simulink model "Voltage_Vector_with_script_fianl"  (R2024b)
settings: Solver=FixedStepAuto  StartTime=0.0  StopTime=0.5  FixedStep=1e-5  RelTol=1e-3
model workspace (MAT data in the model file):
  Cap = 0.004
  FL = 0.025
  Indcut = 0.005
  Initial_Voltage = 125
  R_Load = 1000
  V_dc = 300
  Vd = 125
  Vl = 400
  c = 125
  cap = 7.07e-05
  f_o = 50
  f_s = 5000
libraries: spsIGBTDiodeLib x72, spsSeriesRLCBranchLib x48, spsMultimeterLib x9, spsRMSLib x7, spsThreePhaseBreakerLib x6, spsTHDLib x6, spsThreePhaseSeriesRLCLoadLib x4, spsGroundLib x3, spsCurrentMeasurementLib x2, spsDCVoltageSourceLib x2, spsThreePhaseVIMeasurementLib x2, slpidlib x1
(part 2 of 3)

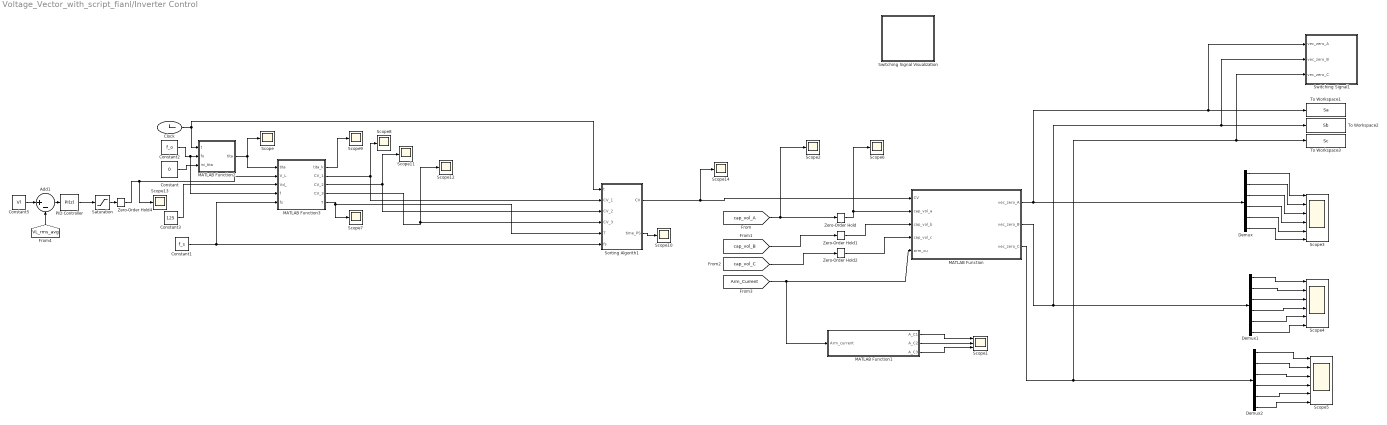
== system Voltage_Vector_with_script_fianl/Inverter Control ==
  Add1 : Sum  Inputs=|+-
  Clock : Clock
  Constant : Constant  Value=0
  Constant1 : Constant  Value=f_s
  Constant2 : Constant  Value=f_o
  Constant3 : Constant  Value=125
  Constant5 : Constant  Value=Vl
  Demux : Demux  Outputs=6
  Demux1 : Demux  Outputs=6
  Demux2 : Demux  Outputs=6
  MATLAB Function : MATLAB Function  TreatAsAtomicUnit=on
  MATLAB Function1 : MATLAB Function  TreatAsAtomicUnit=on
  MATLAB Function2 : MATLAB Function  TreatAsAtomicUnit=on
  MATLAB Function3 : MATLAB Function  TreatAsAtomicUnit=on
  PID Controller : slpidlib/PID Controller  Controller=PI  Form=Parallel  TimeDomain=Discrete-time  UseExternalTs=off  SampleTime=-1  IntegratorMethod=Forward Euler  FilterMethod=Forward Euler  ControllerParametersSource=internal  P=9  I=80  UseKiTs=off  D=0  UseExternalDerivativeSource=off  N=100  UseFilter=on  TunerSelectOption=Transfer Function Based (PID Tuner App)  InitialConditionSource=internal  InitialConditionForIntegrator=0  InitialConditionForFilter=0  DifferentiatorICPrevScaledInput=0  ExternalReset=none  TrackingMode=off  Kt=1  LimitOutput=off  SatLimitsSource=internal  UpperSaturationLimit=inf  LowerSaturationLimit=-inf  LinearizeAsGain=on  AntiWindupMode=none  Kb=1  LimitIntegrator=off  UpperIntegratorSaturationLimit=inf  LowerIntegratorSaturationLimit=-inf  POutMin=[]  POutMax=[]  IOutMin=[]  IOutMax=[]  DOutMin=[]  DOutMax=[]  NOutMin=[]  NOutMax=[]  SumOutMin=[]  SumOutMax=[]  SaturationOutMin=[]  SaturationOutMax=[]  PParamMin=[]  PParamMax=[]  IParamMin=[]  IParamMax=[]  DParamMin=[]  DParamMax=[]  NParamMin=[]  NParamMax=[]  KbParamMin=[]  KbParamMax=[]  KtParamMin=[]  KtParamMax=[]  KbOutMin=[]  KbOutMax=[]  KtOutMin=[]  KtOutMax=[]  IntegratorOutMin=[]  IntegratorOutMax=[]  FilterOutMin=[]  FilterOutMax=[]  SumI1OutMin=[]  SumI1OutMax=[]  SumI2OutMin=[]  SumI2OutMax=[]  SumI3OutMin=[]  SumI3OutMax=[]  SumI4OutMin=[]  SumI4OutMax=[]  SumDOutMin=[]  SumDOutMax=[]  DifferentiatorOutMin=[]  DifferentiatorOutMax=[]  FilterDiffOutCoefMin=[]  FilterDiffOutCoefMax=[]  ReciprocalOutMin=[]  ReciprocalOutMax=[]  SumDenOutMin=[]  SumDenOutMax=[]  SumNumOutMin=[]  SumNumOutMax=[]  DivideOutMin=[]  DivideOutMax=[]  UdiffTsProdOutMin=[]  UdiffTsProdOutMax=[]  NTsProdOutMin=[]  NTsProdOutMax=[]  UintegralTsProdOutMin=[]  UintegralTsProdOutMax=[]  UngainTsProdOutMin=[]  UngainTsProdOutMax=[]  ClampingZeroOutDataTypeStr=Inherit: Inherit via back propagation  ClampingZeroOutMin=[]  ClampingZeroOutMax=[]  FilterDenConstantOutDataTypeStr=Inherit: Inherit via back propagation  FilterDenConstantOutMin=[]  FilterDenConstantOutMax=[]  PCopyOutDataTypeStr=Inherit: Inherit via back propagation  PCopyOutMin=[]  PCopyOutMax=[]  NCopyOutDataTypeStr=Inherit: Inherit via back propagation  NCopyOutMin=[]  NCopyOutMax=[]  IntegratorContinuousStateAttributes=''  IntegratorStateMustResolveToSignalObject=off  IntegratorRTWStateStorageClass=Auto  FilterContinuousStateAttributes=''  FilterStateMustResolveToSignalObject=off  FilterRTWStateStorageClass=Auto  ParallelPVariant=InternalParameters  IdealPVariant=Disabled  IVariant=InternalParameters  DVariant=Disabled  IntegratorVariant=Discrete  SatVariant=Disabled  AWVariant=Passthrough  PCopyVariant=Disabled  TRVariant=Disabled  FdbkBlocksVariant=Forward  IdealPFdbkVariant=Disabled  SatFdbkVariant=Disabled  DerivativeFilterVariant=Disabled  NVariant=Disabled  NCopyVariant=Disabled_SignalSpec  FilterICVariant=Disabled  IntegratorICVariant=InternalICs  ExternalResetVariant=Disabled  TRSumVariant=Passthrough  SumFdbkVariant=Disabled  SumVariant=Sum_PI  TsampFilterVariant=InternalTs  TsampNgainVariant=Passthrough  TsampIntegralVariant=Disabled_SignalSpec  ExternalSaturationOutDataTypeStr=Inherit: Same as second input  DerivativeSourceVariant=Disabled  PreIntVariant=InternalPreInt
  Saturation : Saturate  UpperLimit=450  LowerLimit=350
  Scope{,2,6..14} (11 alike) : Scope
  Scope1 : Scope  NumInputPorts=3
  Scope3 : Scope  NumInputPorts=6
  Scope4 : Scope  NumInputPorts=6
  Scope5 : Scope  NumInputPorts=6
  Sorting Algorith1 : MATLAB Function  TreatAsAtomicUnit=on
  Switching Signal Visualization : Subsystem
  Switching Signal1 : Subsystem
  To Workspace1 : ToWorkspace  VariableName=Sa  SaveFormat=Timeseries  SampleTime=-1
      settings: Decimation=10
  To Workspace2 : ToWorkspace  VariableName=Sb  SaveFormat=Timeseries  SampleTime=-1
  To Workspace3 : ToWorkspace  VariableName=Sc  SaveFormat=Timeseries  SampleTime=-1
  Zero-Order Hold{,1..2,4} (4 alike) : ZeroOrderHold  SampleTime=1/5000
  wires:
  [cap_vol_A] -> Zero-Order Hold/1, Scope2/1
  [Arm_Current] -> MATLAB Function/5(arm_cu), MATLAB Function1/1(Arm_current)
  MATLAB Function1/1(A_C1) -> Scope1/1
  MATLAB Function1/2(A_C2) -> Scope1/2
  MATLAB Function1/3(A_C3) -> Scope1/3
  Demux2/1 -> Scope5/1
  Demux2/6 -> Scope5/6
  Demux2/2 -> Scope5/2
  Demux2/3 -> Scope5/3
  Demux2/4 -> Scope5/4
  Demux2/5 -> Scope5/5
  Demux1/1 -> Scope4/1
  Demux1/6 -> Scope4/6
  Demux1/2 -> Scope4/2
  Demux1/3 -> Scope4/3
  Demux1/4 -> Scope4/4
  Demux1/5 -> Scope4/5
  MATLAB Function/2(vec_zero_B) -> Switching Signal1/2(vec_zero_B), To Workspace2/1, Demux1/1
  Demux/6 -> Scope3/6
  Demux/5 -> Scope3/5
  Demux/4 -> Scope3/4
  Demux/3 -> Scope3/3
  Demux/2 -> Scope3/2
  Demux/1 -> Scope3/1
  MATLAB Function/1(vec_zero_A) -> Switching Signal1/1(vec_zero_A), To Workspace1/1, Demux/1
  MATLAB Function/3(vec_zero_C) -> Switching Signal1/3(vec_zero_C), To Workspace3/1, Demux2/1
  Zero-Order Hold/1 -> Scope6/1, MATLAB Function/2(cap_vol_a)
  [cap_vol_B] -> Zero-Order Hold1/1
  Zero-Order Hold1/1 -> MATLAB Function/3(cap_vol_b)
  [cap_vol_C] -> Zero-Order Hold2/1
  Zero-Order Hold2/1 -> MATLAB Function/4(cap_vol_c)
  MATLAB Function3/4(CV_3) -> Scope12/1, Sorting Algorith1/4(CV_3)
  MATLAB Function3/3(CV_2) -> Scope11/1, Sorting Algorith1/3(CV_2)
  MATLAB Function3/5(T) -> Scope7/1, Sorting Algorith1/5(T)
  MATLAB Function3/1(tita_k) -> Scope9/1
  Constant2/1 -> MATLAB Function3/4(f), MATLAB Function2/2(fo)
  MATLAB Function2/1(tita) -> MATLAB Function3/1(tita), Scope/1
  Constant/1 -> MATLAB Function2/3(ini_tita)
  MATLAB Function3/2(CV_1) -> Scope8/1, Sorting Algorith1/2(CV_1)
  Clock/1 -> MATLAB Function2/1(t), Sorting Algorith1/1(t)
  Sorting Algorith1/1(CV) -> Scope14/1, MATLAB Function/1(CV)
  Sorting Algorith1/2(time_PS) -> Scope10/1
  Constant1/1 -> MATLAB Function3/5(fs), Sorting Algorith1/6(fs)
  Constant3/1 -> MATLAB Function3/3(Vd_)
  Constant5/1 -> Add1/1
  [VL_rms_avg] -> Add1/2
  Add1/1 -> PID Controller/1
  PID Controller/1 -> Saturation/1
  Saturation/1 -> Zero-Order Hold4/1
  Zero-Order Hold4/1 -> Scope13/1, MATLAB Function3/2(V_L)

== system Voltage_Vector_with_script_fianl/LC Filter ==
  Ground : spsGroundLib/Ground  LConnTagsString=a
  Series RLC Branch : spsSeriesRLCBranchLib/Series RLC Branch  LConnTagsString=__new0  RConnTagsString=__new0  BranchType=L  Resistance=1  Inductance=FL  SetiL0=off  InitialCurrent=0  Capacitance=1e-6  Setx0=off  InitialVoltage=0  Measurements=None
  Series RLC Branch1 : spsSeriesRLCBranchLib/Series RLC Branch  LConnTagsString=__new0  RConnTagsString=__new0  BranchType=C  Resistance=1  Inductance=1e-3  SetiL0=off  InitialCurrent=0  Capacitance=cap  Setx0=off  InitialVoltage=0  Measurements=None
  Series RLC Branch2 : spsSeriesRLCBranchLib/Series RLC Branch  LConnTagsString=__new0  RConnTagsString=__new0  BranchType=L  Resistance=1  Inductance=FL  SetiL0=off  InitialCurrent=0  Capacitance=1e-6  Setx0=off  InitialVoltage=0  Measurements=None
  Series RLC Branch3 : spsSeriesRLCBranchLib/Series RLC Branch  LConnTagsString=__new0  RConnTagsString=__new0  BranchType=L  Resistance=1  Inductance=FL  SetiL0=off  InitialCurrent=0  Capacitance=1e-6  Setx0=off  InitialVoltage=0  Measurements=None
  Series RLC Branch4 : spsSeriesRLCBranchLib/Series RLC Branch  LConnTagsString=__new0  RConnTagsString=__new0  BranchType=C  Resistance=1  Inductance=1e-3  SetiL0=off  InitialCurrent=0  Capacitance=cap  Setx0=off  InitialVoltage=0  Measurements=None
  Series RLC Branch5 : spsSeriesRLCBranchLib/Series RLC Branch  LConnTagsString=__new0  RConnTagsString=__new0  BranchType=C  Resistance=1  Inductance=1e-3  SetiL0=off  InitialCurrent=0  Capacitance=cap  Setx0=off  InitialVoltage=0  Measurements=None
  Va in : PMIOPort  Side=Left
  Vb in : PMIOPort  Port=2  Side=Left
  Vc in : PMIOPort  Port=3  Side=Left
  Va out : PMIOPort  Port=4  Side=Right
  Vb out : PMIOPort  Port=5  Side=Right
  Vc out : PMIOPort  Port=6  Side=Right
  connections:
  Va in/RConn1 -- Series RLC Branch/LConn1
  Series RLC Branch2/LConn1 -- Vb in/RConn1
  Vc in/RConn1 -- Series RLC Branch3/LConn1
  Series RLC Branch4/RConn1 -- Ground/LConn1 -- Series RLC Branch1/RConn1 -- Series RLC Branch5/RConn1
  Series RLC Branch4/LConn1 -- Vb out/RConn1 -- Series RLC Branch2/RConn1
  Series RLC Branch/RConn1 -- Va out/RConn1 -- Series RLC Branch1/LConn1
  Series RLC Branch5/LConn1 -- Vc out/RConn1 -- Series RLC Branch3/RConn1

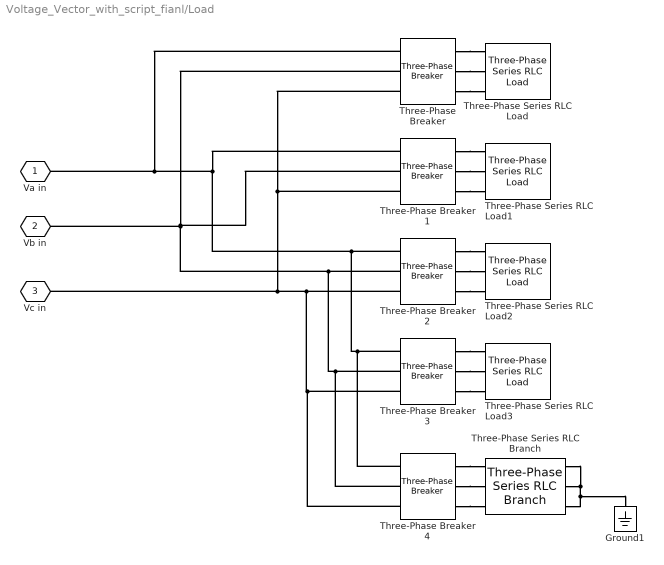
== system Voltage_Vector_with_script_fianl/Load ==
  Ground1 : spsGroundLib/Ground  LConnTagsString=a
  Three-Phase Series RLC Branch : spsThreePhaseSeriesRLCBranchLib/Three-Phase Series RLC Branch  LConnTagsString=A|B|C  RConnTagsString=A|B|C  BranchType=R  Resistance=15  Inductance=1e-3  Capacitance=1e-6  Measurements=None
  Three-Phase Series RLC Load : spsThreePhaseSeriesRLCLoadLib/Three-Phase Series RLC Load  LConnTagsString=A|B|C  Configuration=Y (grounded)  NominalVoltage=400  Vabc=[1e3 1e3 1e3]  Vabcp=[1e3 1e3 1e3]  NominalFrequency=50  UnbalancedPower=off  ActivePower=10000  InductivePower=0  CapacitivePower=0  Pabc=[10e3 9e3 11e3]  QLabc=[100 90 110]  QCabc=[100 90 110]  Pabcp=[10e3 9e3 11e3]  QLabcp=[100 90 110]  QCabcp=[100 90 110]  Measurements=None  LoadType=constant Z
  Three-Phase Series RLC Load1 : spsThreePhaseSeriesRLCLoadLib/Three-Phase Series RLC Load  LConnTagsString=A|B|C  Configuration=Y (grounded)  NominalVoltage=1000  Vabc=[1e3 1e3 1e3]  Vabcp=[1e3 1e3 1e3]  NominalFrequency=60  UnbalancedPower=off  ActivePower=10e3  InductivePower=100  CapacitivePower=100  Pabc=[10e3 9e3 11e3]  QLabc=[100 90 110]  QCabc=[100 90 110]  Pabcp=[10e3 9e3 11e3]  QLabcp=[100 90 110]  QCabcp=[100 90 110]  Measurements=None  LoadType=constant Z
  Three-Phase Series RLC Load2 : spsThreePhaseSeriesRLCLoadLib/Three-Phase Series RLC Load  LConnTagsString=A|B|C  Configuration=Y (grounded)  NominalVoltage=1000  Vabc=[1e3 1e3 1e3]  Vabcp=[1e3 1e3 1e3]  NominalFrequency=60  UnbalancedPower=off  ActivePower=10e3  InductivePower=100  CapacitivePower=100  Pabc=[10e3 9e3 11e3]  QLabc=[100 90 110]  QCabc=[100 90 110]  Pabcp=[10e3 9e3 11e3]  QLabcp=[100 90 110]  QCabcp=[100 90 110]  Measurements=None  LoadType=constant Z
  Three-Phase Series RLC Load3 : spsThreePhaseSeriesRLCLoadLib/Three-Phase Series RLC Load  LConnTagsString=A|B|C  Configuration=Y (grounded)  NominalVoltage=1000  Vabc=[1e3 1e3 1e3]  Vabcp=[1e3 1e3 1e3]  NominalFrequency=60  UnbalancedPower=off  ActivePower=10e3  InductivePower=100  CapacitivePower=100  Pabc=[10e3 9e3 11e3]  QLabc=[100 90 110]  QCabc=[100 90 110]  Pabcp=[10e3 9e3 11e3]  QLabcp=[100 90 110]  QCabcp=[100 90 110]  Measurements=None  LoadType=constant Z
  Three-Phase Breaker {,1..3} (4 alike) : spsThreePhaseBreakerLib/Three-Phase Breaker  InitialState=open  SwitchA=on  SwitchB=on  SwitchC=on  SwitchTimes="[1/60  5/60]"  External=off  BreakerResistance=0.01  SnubberResistance=1e6  SnubberCapacitance=inf  Measurements=None
  Three-Phase Breaker 4 : spsThreePhaseBreakerLib/Three-Phase Breaker  InitialState=closed  SwitchA=on  SwitchB=on  SwitchC=on  SwitchTimes="[1/60  5/60]"  External=off  BreakerResistance=0.01  SnubberResistance=inf  SnubberCapacitance=inf  Measurements=None
  Va in : PMIOPort  Side=Left
  Vb in : PMIOPort  Port=2  Side=Left
  Vc in : PMIOPort  Port=3  Side=Left
  connections:
  "Three-Phase Breaker "/LConn1 -- Va in/RConn1 -- Three-Phase Breaker 4/LConn1 -- Three-Phase Breaker 3/LConn1 -- Three-Phase Breaker 2/LConn1 -- Three-Phase Breaker 1/LConn1
  "Three-Phase Breaker "/LConn2 -- Three-Phase Breaker 4/LConn2 -- Three-Phase Breaker 3/LConn2 -- Three-Phase Breaker 2/LConn2 -- Vb in/RConn1 -- Three-Phase Breaker 1/LConn2
  Three-Phase Breaker 1/LConn3 -- Vc in/RConn1 -- Three-Phase Breaker 4/LConn3 -- Three-Phase Breaker 3/LConn3 -- Three-Phase Breaker 2/LConn3 -- "Three-Phase Breaker "/LConn3
  "Three-Phase Breaker "/RConn2 -- Three-Phase Series RLC Load/LConn2
  "Three-Phase Breaker "/RConn1 -- Three-Phase Series RLC Load/LConn1
  "Three-Phase Breaker "/RConn3 -- Three-Phase Series RLC Load/LConn3
  Three-Phase Breaker 1/RConn2 -- Three-Phase Series RLC Load1/LConn2
  Three-Phase Breaker 1/RConn3 -- Three-Phase Series RLC Load1/LConn3
  Three-Phase Breaker 1/RConn1 -- Three-Phase Series RLC Load1/LConn1
  Three-Phase Breaker 2/RConn1 -- Three-Phase Series RLC Load2/LConn1
  Three-Phase Breaker 2/RConn3 -- Three-Phase Series RLC Load2/LConn3
  Three-Phase Breaker 2/RConn2 -- Three-Phase Series RLC Load2/LConn2
  Three-Phase Breaker 3/RConn2 -- Three-Phase Series RLC Load3/LConn2
  Three-Phase Breaker 3/RConn3 -- Three-Phase Series RLC Load3/LConn3
  Three-Phase Breaker 3/RConn1 -- Three-Phase Series RLC Load3/LConn1
  Three-Phase Series RLC Branch/RConn1 -- Three-Phase Series RLC Branch/RConn3 -- Ground1/LConn1 -- Three-Phase Series RLC Branch/RConn2
  Three-Phase Breaker 4/RConn1 -- Three-Phase Series RLC Branch/LConn1
  Three-Phase Breaker 4/RConn2 -- Three-Phase Series RLC Branch/LConn2
  Three-Phase Breaker 4/RConn3 -- Three-Phase Series RLC Branch/LConn3

== system Voltage_Vector_with_script_fianl/Measurement ==
  Cap Balancing Signals : Subsystem
  Current Measurements : Subsystem
  Voltage Measurements : Subsystem

== system Voltage_Vector_with_script_fianl/3 ph 7 level MMI/SM 1 phase A ==
  Input : Inport
  IGBT/Diode : spsIGBTDiodeLib/IGBT//Diode  Ron=1e-3  Rs=1e5  Cs=inf  Measurements=on
  IGBT/Diode1 : spsIGBTDiodeLib/IGBT//Diode  Ron=1e-3  Rs=1e5  Cs=inf  Measurements=on
  NOT1 : Logic  Operator=NOT  IconShape=distinctive  AllPortsSameDT=off  OutDataTypeStr=boolean
  Scope : Scope
  Scope1 : Scope
  Scope2 : Scope
  Series RLC Branch2 : spsSeriesRLCBranchLib/Series RLC Branch  LConnTagsString=__new0  RConnTagsString=__new0  BranchType=C  Resistance=1  Inductance=1e-3  SetiL0=off  InitialCurrent=0  Capacitance=Cap  Setx0=on  InitialVoltage=Initial_Voltage  Measurements=Branch voltage and current
  + : PMIOPort  Side=Left
  - : PMIOPort  Port=2  Side=Right
  wires:
  Input/1 -> Scope2/1, IGBT/Diode/1, NOT1/1
  NOT1/1 -> IGBT/Diode1/1
  IGBT/Diode/1 -> Scope/1
  IGBT/Diode1/1 -> Scope1/1
  connections:
  IGBT/Diode1/LConn1 -- IGBT/Diode/RConn1 -- +/RConn1
  Series RLC Branch2/LConn1 -- IGBT/Diode/LConn1
  Series RLC Branch2/RConn1 -- -/RConn1 -- IGBT/Diode1/RConn1

== system Voltage_Vector_with_script_fianl/3 ph 7 level MMI/SM 1 phase B ==
  Input : Inport
  IGBT/Diode : spsIGBTDiodeLib/IGBT//Diode  Ron=1e-3  Rs=1e5  Cs=inf  Measurements=on
  IGBT/Diode1 : spsIGBTDiodeLib/IGBT//Diode  Ron=1e-3  Rs=1e5  Cs=inf  Measurements=on
  NOT1 : Logic  Operator=NOT  IconShape=distinctive  AllPortsSameDT=off  OutDataTypeStr=boolean
  Series RLC Branch2 : spsSeriesRLCBranchLib/Series RLC Branch  LConnTagsString=__new0  RConnTagsString=__new0  BranchType=C  Resistance=1  Inductance=1e-3  SetiL0=off  InitialCurrent=0  Capacitance=Cap  Setx0=on  InitialVoltage=Initial_Voltage  Measurements=Branch voltage and current
  + : PMIOPort  Side=Left
  - : PMIOPort  Port=2  Side=Right
  wires:
  Input/1 -> IGBT/Diode/1, NOT1/1
  NOT1/1 -> IGBT/Diode1/1
  connections:
  +/RConn1 -- IGBT/Diode1/LConn1 -- IGBT/Diode/RConn1
  Series RLC Branch2/LConn1 -- IGBT/Diode/LConn1
  Series RLC Branch2/RConn1 -- -/RConn1 -- IGBT/Diode1/RConn1

== system Voltage_Vector_with_script_fianl/3 ph 7 level MMI/SM 1 phase C ==
  Input : Inport
  IGBT/Diode : spsIGBTDiodeLib/IGBT//Diode  Ron=1e-3  Rs=1e5  Cs=inf  Measurements=on
  IGBT/Diode1 : spsIGBTDiodeLib/IGBT//Diode  Ron=1e-3  Rs=1e5  Cs=inf  Measurements=on
  NOT1 : Logic  Operator=NOT  IconShape=distinctive  AllPortsSameDT=off  OutDataTypeStr=boolean
  Series RLC Branch2 : spsSeriesRLCBranchLib/Series RLC Branch  LConnTagsString=__new0  RConnTagsString=__new0  BranchType=C  Resistance=1  Inductance=1e-3  SetiL0=off  InitialCurrent=0  Capacitance=Cap  Setx0=on  InitialVoltage=Initial_Voltage  Measurements=Branch voltage and current
  + : PMIOPort  Side=Left
  - : PMIOPort  Port=2  Side=Right
  wires:
  Input/1 -> IGBT/Diode/1, NOT1/1
  NOT1/1 -> IGBT/Diode1/1
  connections:
  +/RConn1 -- IGBT/Diode1/LConn1 -- IGBT/Diode/RConn1
  Series RLC Branch2/LConn1 -- IGBT/Diode/LConn1
  Series RLC Branch2/RConn1 -- -/RConn1 -- IGBT/Diode1/RConn1

== system Voltage_Vector_with_script_fianl/3 ph 7 level MMI/SM 10 phase A ==
  Input : Inport
  IGBT/Diode : spsIGBTDiodeLib/IGBT//Diode  Ron=1e-3  Rs=1e5  Cs=inf  Measurements=on
  IGBT/Diode1 : spsIGBTDiodeLib/IGBT//Diode  Ron=1e-3  Rs=1e5  Cs=inf  Measurements=on
  NOT1 : Logic  Operator=NOT  IconShape=distinctive  AllPortsSameDT=off  OutDataTypeStr=boolean
  Series RLC Branch2 : spsSeriesRLCBranchLib/Series RLC Branch  LConnTagsString=__new0  RConnTagsString=__new0  BranchType=C  Resistance=1  Inductance=1e-3  SetiL0=off  InitialCurrent=0  Capacitance=Cap  Setx0=on  InitialVoltage=Initial_Voltage  Measurements=Branch voltage and current
  + : PMIOPort  Side=Left
  - : PMIOPort  Port=2  Side=Right
  wires:
  Input/1 -> IGBT/Diode/1, NOT1/1
  NOT1/1 -> IGBT/Diode1/1
  connections:
  +/RConn1 -- IGBT/Diode1/LConn1 -- IGBT/Diode/RConn1
  Series RLC Branch2/LConn1 -- IGBT/Diode/LConn1
  Series RLC Branch2/RConn1 -- -/RConn1 -- IGBT/Diode1/RConn1

== system Voltage_Vector_with_script_fianl/3 ph 7 level MMI/SM 10 phase B ==
  Input : Inport
  IGBT/Diode : spsIGBTDiodeLib/IGBT//Diode  Ron=1e-3  Rs=1e5  Cs=inf  Measurements=on
  IGBT/Diode1 : spsIGBTDiodeLib/IGBT//Diode  Ron=1e-3  Rs=1e5  Cs=inf  Measurements=on
  NOT1 : Logic  Operator=NOT  IconShape=distinctive  AllPortsSameDT=off  OutDataTypeStr=boolean
  Series RLC Branch2 : spsSeriesRLCBranchLib/Series RLC Branch  LConnTagsString=__new0  RConnTagsString=__new0  BranchType=C  Resistance=1  Inductance=1e-3  SetiL0=off  InitialCurrent=0  Capacitance=Cap  Setx0=on  InitialVoltage=Initial_Voltage  Measurements=Branch voltage and current
  + : PMIOPort  Side=Left
  - : PMIOPort  Port=2  Side=Right
  wires:
  Input/1 -> IGBT/Diode/1, NOT1/1
  NOT1/1 -> IGBT/Diode1/1
  connections:
  +/RConn1 -- IGBT/Diode1/LConn1 -- IGBT/Diode/RConn1
  Series RLC Branch2/LConn1 -- IGBT/Diode/LConn1
  Series RLC Branch2/RConn1 -- -/RConn1 -- IGBT/Diode1/RConn1

== system Voltage_Vector_with_script_fianl/3 ph 7 level MMI/SM 10 phase C ==
  Input : Inport
  IGBT/Diode : spsIGBTDiodeLib/IGBT//Diode  Ron=1e-3  Rs=1e5  Cs=inf  Measurements=on
  IGBT/Diode1 : spsIGBTDiodeLib/IGBT//Diode  Ron=1e-3  Rs=1e5  Cs=inf  Measurements=on
  NOT1 : Logic  Operator=NOT  IconShape=distinctive  AllPortsSameDT=off  OutDataTypeStr=boolean
  Series RLC Branch2 : spsSeriesRLCBranchLib/Series RLC Branch  LConnTagsString=__new0  RConnTagsString=__new0  BranchType=C  Resistance=1  Inductance=1e-3  SetiL0=off  InitialCurrent=0  Capacitance=Cap  Setx0=on  InitialVoltage=Initial_Voltage  Measurements=Branch voltage and current
  + : PMIOPort  Side=Left
  - : PMIOPort  Port=2  Side=Right
  wires:
  Input/1 -> IGBT/Diode/1, NOT1/1
  NOT1/1 -> IGBT/Diode1/1
  connections:
  +/RConn1 -- IGBT/Diode1/LConn1 -- IGBT/Diode/RConn1
  Series RLC Branch2/LConn1 -- IGBT/Diode/LConn1
  Series RLC Branch2/RConn1 -- -/RConn1 -- IGBT/Diode1/RConn1

== system Voltage_Vector_with_script_fianl/3 ph 7 level MMI/SM 11 phase A ==
  Input : Inport
  IGBT/Diode : spsIGBTDiodeLib/IGBT//Diode  Ron=1e-3  Rs=1e5  Cs=inf  Measurements=on
  IGBT/Diode1 : spsIGBTDiodeLib/IGBT//Diode  Ron=1e-3  Rs=1e5  Cs=inf  Measurements=on
  NOT1 : Logic  Operator=NOT  IconShape=distinctive  AllPortsSameDT=off  OutDataTypeStr=boolean
  Series RLC Branch2 : spsSeriesRLCBranchLib/Series RLC Branch  LConnTagsString=__new0  RConnTagsString=__new0  BranchType=C  Resistance=1  Inductance=1e-3  SetiL0=off  InitialCurrent=0  Capacitance=Cap  Setx0=on  InitialVoltage=Initial_Voltage  Measurements=Branch voltage and current
  + : PMIOPort  Side=Left
  - : PMIOPort  Port=2  Side=Right
  wires:
  Input/1 -> IGBT/Diode/1, NOT1/1
  NOT1/1 -> IGBT/Diode1/1
  connections:
  +/RConn1 -- IGBT/Diode1/LConn1 -- IGBT/Diode/RConn1
  Series RLC Branch2/LConn1 -- IGBT/Diode/LConn1
  Series RLC Branch2/RConn1 -- -/RConn1 -- IGBT/Diode1/RConn1

== system Voltage_Vector_with_script_fianl/3 ph 7 level MMI/SM 11 phase B ==
  Input : Inport
  IGBT/Diode : spsIGBTDiodeLib/IGBT//Diode  Ron=1e-3  Rs=1e5  Cs=inf  Measurements=on
  IGBT/Diode1 : spsIGBTDiodeLib/IGBT//Diode  Ron=1e-3  Rs=1e5  Cs=inf  Measurements=on
  NOT1 : Logic  Operator=NOT  IconShape=distinctive  AllPortsSameDT=off  OutDataTypeStr=boolean
  Series RLC Branch2 : spsSeriesRLCBranchLib/Series RLC Branch  LConnTagsString=__new0  RConnTagsString=__new0  BranchType=C  Resistance=1  Inductance=1e-3  SetiL0=off  InitialCurrent=0  Capacitance=Cap  Setx0=on  InitialVoltage=Initial_Voltage  Measurements=Branch voltage and current
  + : PMIOPort  Side=Left
  - : PMIOPort  Port=2  Side=Right
  wires:
  Input/1 -> IGBT/Diode/1, NOT1/1
  NOT1/1 -> IGBT/Diode1/1
  connections:
  +/RConn1 -- IGBT/Diode1/LConn1 -- IGBT/Diode/RConn1
  Series RLC Branch2/LConn1 -- IGBT/Diode/LConn1
  Series RLC Branch2/RConn1 -- -/RConn1 -- IGBT/Diode1/RConn1

== system Voltage_Vector_with_script_fianl/3 ph 7 level MMI/SM 11 phase C ==
  Input : Inport
  IGBT/Diode : spsIGBTDiodeLib/IGBT//Diode  Ron=1e-3  Rs=1e5  Cs=inf  Measurements=on
  IGBT/Diode1 : spsIGBTDiodeLib/IGBT//Diode  Ron=1e-3  Rs=1e5  Cs=inf  Measurements=on
  NOT1 : Logic  Operator=NOT  IconShape=distinctive  AllPortsSameDT=off  OutDataTypeStr=boolean
  Series RLC Branch2 : spsSeriesRLCBranchLib/Series RLC Branch  LConnTagsString=__new0  RConnTagsString=__new0  BranchType=C  Resistance=1  Inductance=1e-3  SetiL0=off  InitialCurrent=0  Capacitance=Cap  Setx0=on  InitialVoltage=Initial_Voltage  Measurements=Branch voltage and current
  + : PMIOPort  Side=Left
  - : PMIOPort  Port=2  Side=Right
  wires:
  Input/1 -> IGBT/Diode/1, NOT1/1
  NOT1/1 -> IGBT/Diode1/1
  connections:
  +/RConn1 -- IGBT/Diode1/LConn1 -- IGBT/Diode/RConn1
  Series RLC Branch2/LConn1 -- IGBT/Diode/LConn1
  Series RLC Branch2/RConn1 -- -/RConn1 -- IGBT/Diode1/RConn1

== system Voltage_Vector_with_script_fianl/3 ph 7 level MMI/SM 12 phase A ==
  Input : Inport
  IGBT/Diode : spsIGBTDiodeLib/IGBT//Diode  Ron=1e-3  Rs=1e5  Cs=inf  Measurements=on
  IGBT/Diode1 : spsIGBTDiodeLib/IGBT//Diode  Ron=1e-3  Rs=1e5  Cs=inf  Measurements=on
  NOT1 : Logic  Operator=NOT  IconShape=distinctive  AllPortsSameDT=off  OutDataTypeStr=boolean
  Series RLC Branch2 : spsSeriesRLCBranchLib/Series RLC Branch  LConnTagsString=__new0  RConnTagsString=__new0  BranchType=C  Resistance=1  Inductance=1e-3  SetiL0=off  InitialCurrent=0  Capacitance=Cap  Setx0=on  InitialVoltage=Initial_Voltage  Measurements=Branch voltage and current
  + : PMIOPort  Side=Left
  - : PMIOPort  Port=2  Side=Right
  wires:
  Input/1 -> IGBT/Diode/1, NOT1/1
  NOT1/1 -> IGBT/Diode1/1
  connections:
  +/RConn1 -- IGBT/Diode1/LConn1 -- IGBT/Diode/RConn1
  Series RLC Branch2/LConn1 -- IGBT/Diode/LConn1
  Series RLC Branch2/RConn1 -- -/RConn1 -- IGBT/Diode1/RConn1

== system Voltage_Vector_with_script_fianl/3 ph 7 level MMI/SM 12 phase B ==
  Input : Inport
  IGBT/Diode : spsIGBTDiodeLib/IGBT//Diode  Ron=1e-3  Rs=1e5  Cs=inf  Measurements=on
  IGBT/Diode1 : spsIGBTDiodeLib/IGBT//Diode  Ron=1e-3  Rs=1e5  Cs=inf  Measurements=on
  NOT1 : Logic  Operator=NOT  IconShape=distinctive  AllPortsSameDT=off  OutDataTypeStr=boolean
  Series RLC Branch2 : spsSeriesRLCBranchLib/Series RLC Branch  LConnTagsString=__new0  RConnTagsString=__new0  BranchType=C  Resistance=1  Inductance=1e-3  SetiL0=off  InitialCurrent=0  Capacitance=Cap  Setx0=on  InitialVoltage=Initial_Voltage  Measurements=Branch voltage and current
  + : PMIOPort  Side=Left
  - : PMIOPort  Port=2  Side=Right
  wires:
  Input/1 -> IGBT/Diode/1, NOT1/1
  NOT1/1 -> IGBT/Diode1/1
  connections:
  +/RConn1 -- IGBT/Diode1/LConn1 -- IGBT/Diode/RConn1
  Series RLC Branch2/LConn1 -- IGBT/Diode/LConn1
  Series RLC Branch2/RConn1 -- -/RConn1 -- IGBT/Diode1/RConn1

== system Voltage_Vector_with_script_fianl/3 ph 7 level MMI/SM 12 phase C ==
  Input : Inport
  IGBT/Diode : spsIGBTDiodeLib/IGBT//Diode  Ron=1e-3  Rs=1e5  Cs=inf  Measurements=on
  IGBT/Diode1 : spsIGBTDiodeLib/IGBT//Diode  Ron=1e-3  Rs=1e5  Cs=inf  Measurements=on
  NOT1 : Logic  Operator=NOT  IconShape=distinctive  AllPortsSameDT=off  OutDataTypeStr=boolean
  Series RLC Branch2 : spsSeriesRLCBranchLib/Series RLC Branch  LConnTagsString=__new0  RConnTagsString=__new0  BranchType=C  Resistance=1  Inductance=1e-3  SetiL0=off  InitialCurrent=0  Capacitance=Cap  Setx0=on  InitialVoltage=Initial_Voltage  Measurements=Branch voltage and current
  + : PMIOPort  Side=Left
  - : PMIOPort  Port=2  Side=Right
  wires:
  Input/1 -> IGBT/Diode/1, NOT1/1
  NOT1/1 -> IGBT/Diode1/1
  connections:
  +/RConn1 -- IGBT/Diode1/LConn1 -- IGBT/Diode/RConn1
  Series RLC Branch2/LConn1 -- IGBT/Diode/LConn1
  Series RLC Branch2/RConn1 -- -/RConn1 -- IGBT/Diode1/RConn1

== system Voltage_Vector_with_script_fianl/3 ph 7 level MMI/SM 2 phase A ==
  Input : Inport
  IGBT/Diode : spsIGBTDiodeLib/IGBT//Diode  Ron=1e-3  Rs=1e5  Cs=inf  Measurements=on
  IGBT/Diode1 : spsIGBTDiodeLib/IGBT//Diode  Ron=1e-3  Rs=1e5  Cs=inf  Measurements=on
  NOT1 : Logic  Operator=NOT  IconShape=distinctive  AllPortsSameDT=off  OutDataTypeStr=boolean
  Scope : Scope
  Series RLC Branch2 : spsSeriesRLCBranchLib/Series RLC Branch  LConnTagsString=__new0  RConnTagsString=__new0  BranchType=C  Resistance=1  Inductance=1e-3  SetiL0=off  InitialCurrent=0  Capacitance=Cap  Setx0=on  InitialVoltage=Initial_Voltage  Measurements=Branch voltage and current
  + : PMIOPort  Side=Left
  - : PMIOPort  Port=2  Side=Right
  wires:
  Input/1 -> Scope/1, IGBT/Diode/1, NOT1/1
  NOT1/1 -> IGBT/Diode1/1
  connections:
  +/RConn1 -- IGBT/Diode1/LConn1 -- IGBT/Diode/RConn1
  Series RLC Branch2/LConn1 -- IGBT/Diode/LConn1
  Series RLC Branch2/RConn1 -- -/RConn1 -- IGBT/Diode1/RConn1

== system Voltage_Vector_with_script_fianl/3 ph 7 level MMI/SM 2 phase B ==
  Input : Inport
  IGBT/Diode : spsIGBTDiodeLib/IGBT//Diode  Ron=1e-3  Rs=1e5  Cs=inf  Measurements=on
  IGBT/Diode1 : spsIGBTDiodeLib/IGBT//Diode  Ron=1e-3  Rs=1e5  Cs=inf  Measurements=on
  NOT1 : Logic  Operator=NOT  IconShape=distinctive  AllPortsSameDT=off  OutDataTypeStr=boolean
  Series RLC Branch2 : spsSeriesRLCBranchLib/Series RLC Branch  LConnTagsString=__new0  RConnTagsString=__new0  BranchType=C  Resistance=1  Inductance=1e-3  SetiL0=off  InitialCurrent=0  Capacitance=Cap  Setx0=on  InitialVoltage=Initial_Voltage  Measurements=Branch voltage and current
  + : PMIOPort  Side=Left
  - : PMIOPort  Port=2  Side=Right
  wires:
  Input/1 -> IGBT/Diode/1, NOT1/1
  NOT1/1 -> IGBT/Diode1/1
  connections:
  +/RConn1 -- IGBT/Diode1/LConn1 -- IGBT/Diode/RConn1
  Series RLC Branch2/LConn1 -- IGBT/Diode/LConn1
  Series RLC Branch2/RConn1 -- -/RConn1 -- IGBT/Diode1/RConn1

== system Voltage_Vector_with_script_fianl/3 ph 7 level MMI/SM 2 phase C ==
  Input : Inport
  IGBT/Diode : spsIGBTDiodeLib/IGBT//Diode  Ron=1e-3  Rs=1e5  Cs=inf  Measurements=on
  IGBT/Diode1 : spsIGBTDiodeLib/IGBT//Diode  Ron=1e-3  Rs=1e5  Cs=inf  Measurements=on
  NOT1 : Logic  Operator=NOT  IconShape=distinctive  AllPortsSameDT=off  OutDataTypeStr=boolean
  Series RLC Branch2 : spsSeriesRLCBranchLib/Series RLC Branch  LConnTagsString=__new0  RConnTagsString=__new0  BranchType=C  Resistance=1  Inductance=1e-3  SetiL0=off  InitialCurrent=0  Capacitance=Cap  Setx0=on  InitialVoltage=Initial_Voltage  Measurements=Branch voltage and current
  + : PMIOPort  Side=Left
  - : PMIOPort  Port=2  Side=Right
  wires:
  Input/1 -> IGBT/Diode/1, NOT1/1
  NOT1/1 -> IGBT/Diode1/1
  connections:
  +/RConn1 -- IGBT/Diode1/LConn1 -- IGBT/Diode/RConn1
  Series RLC Branch2/LConn1 -- IGBT/Diode/LConn1
  Series RLC Branch2/RConn1 -- -/RConn1 -- IGBT/Diode1/RConn1

== system Voltage_Vector_with_script_fianl/3 ph 7 level MMI/SM 3 phase A ==
  Input : Inport
  IGBT/Diode : spsIGBTDiodeLib/IGBT//Diode  Ron=1e-3  Rs=1e5  Cs=inf  Measurements=on
  IGBT/Diode1 : spsIGBTDiodeLib/IGBT//Diode  Ron=1e-3  Rs=1e5  Cs=inf  Measurements=on
  NOT1 : Logic  Operator=NOT  IconShape=distinctive  AllPortsSameDT=off  OutDataTypeStr=boolean
  Series RLC Branch2 : spsSeriesRLCBranchLib/Series RLC Branch  LConnTagsString=__new0  RConnTagsString=__new0  BranchType=C  Resistance=1  Inductance=1e-3  SetiL0=off  InitialCurrent=0  Capacitance=Cap  Setx0=on  InitialVoltage=Initial_Voltage  Measurements=Branch voltage and current
  + : PMIOPort  Side=Left
  - : PMIOPort  Port=2  Side=Right
  wires:
  Input/1 -> IGBT/Diode/1, NOT1/1
  NOT1/1 -> IGBT/Diode1/1
  connections:
  +/RConn1 -- IGBT/Diode1/LConn1 -- IGBT/Diode/RConn1
  Series RLC Branch2/LConn1 -- IGBT/Diode/LConn1
  Series RLC Branch2/RConn1 -- -/RConn1 -- IGBT/Diode1/RConn1

== system Voltage_Vector_with_script_fianl/3 ph 7 level MMI/SM 3 phase B ==
  Input : Inport
  IGBT/Diode : spsIGBTDiodeLib/IGBT//Diode  Ron=1e-3  Rs=1e5  Cs=inf  Measurements=on
  IGBT/Diode1 : spsIGBTDiodeLib/IGBT//Diode  Ron=1e-3  Rs=1e5  Cs=inf  Measurements=on
  NOT1 : Logic  Operator=NOT  IconShape=distinctive  AllPortsSameDT=off  OutDataTypeStr=boolean
  Series RLC Branch2 : spsSeriesRLCBranchLib/Series RLC Branch  LConnTagsString=__new0  RConnTagsString=__new0  BranchType=C  Resistance=1  Inductance=1e-3  SetiL0=off  InitialCurrent=0  Capacitance=Cap  Setx0=on  InitialVoltage=Initial_Voltage  Measurements=Branch voltage and current
  + : PMIOPort  Side=Left
  - : PMIOPort  Port=2  Side=Right
  wires:
  Input/1 -> IGBT/Diode/1, NOT1/1
  NOT1/1 -> IGBT/Diode1/1
  connections:
  +/RConn1 -- IGBT/Diode1/LConn1 -- IGBT/Diode/RConn1
  Series RLC Branch2/LConn1 -- IGBT/Diode/LConn1
  Series RLC Branch2/RConn1 -- -/RConn1 -- IGBT/Diode1/RConn1

== system Voltage_Vector_with_script_fianl/3 ph 7 level MMI/SM 3 phase C ==
  Input : Inport
  IGBT/Diode : spsIGBTDiodeLib/IGBT//Diode  Ron=1e-3  Rs=1e5  Cs=inf  Measurements=on
  IGBT/Diode1 : spsIGBTDiodeLib/IGBT//Diode  Ron=1e-3  Rs=1e5  Cs=inf  Measurements=on
  NOT1 : Logic  Operator=NOT  IconShape=distinctive  AllPortsSameDT=off  OutDataTypeStr=boolean
  Series RLC Branch2 : spsSeriesRLCBranchLib/Series RLC Branch  LConnTagsString=__new0  RConnTagsString=__new0  BranchType=C  Resistance=1  Inductance=1e-3  SetiL0=off  InitialCurrent=0  Capacitance=Cap  Setx0=on  InitialVoltage=Initial_Voltage  Measurements=Branch voltage and current
  + : PMIOPort  Side=Left
  - : PMIOPort  Port=2  Side=Right
  wires:
  Input/1 -> IGBT/Diode/1, NOT1/1
  NOT1/1 -> IGBT/Diode1/1
  connections:
  +/RConn1 -- IGBT/Diode1/LConn1 -- IGBT/Diode/RConn1
  Series RLC Branch2/LConn1 -- IGBT/Diode/LConn1
  Series RLC Branch2/RConn1 -- -/RConn1 -- IGBT/Diode1/RConn1

== system Voltage_Vector_with_script_fianl/3 ph 7 level MMI/SM 4 phase A ==
  Input : Inport
  IGBT/Diode : spsIGBTDiodeLib/IGBT//Diode  Ron=1e-3  Rs=1e5  Cs=inf  Measurements=on
  IGBT/Diode1 : spsIGBTDiodeLib/IGBT//Diode  Ron=1e-3  Rs=1e5  Cs=inf  Measurements=on
  NOT1 : Logic  Operator=NOT  IconShape=distinctive  AllPortsSameDT=off  OutDataTypeStr=boolean
  Series RLC Branch2 : spsSeriesRLCBranchLib/Series RLC Branch  LConnTagsString=__new0  RConnTagsString=__new0  BranchType=C  Resistance=1  Inductance=1e-3  SetiL0=off  InitialCurrent=0  Capacitance=Cap  Setx0=on  InitialVoltage=Initial_Voltage  Measurements=Branch voltage and current
  + : PMIOPort  Side=Left
  - : PMIOPort  Port=2  Side=Right
  wires:
  Input/1 -> IGBT/Diode/1, NOT1/1
  NOT1/1 -> IGBT/Diode1/1
  connections:
  +/RConn1 -- IGBT/Diode1/LConn1 -- IGBT/Diode/RConn1
  Series RLC Branch2/LConn1 -- IGBT/Diode/LConn1
  Series RLC Branch2/RConn1 -- -/RConn1 -- IGBT/Diode1/RConn1

== system Voltage_Vector_with_script_fianl/3 ph 7 level MMI/SM 4 phase B ==
  Input : Inport
  IGBT/Diode : spsIGBTDiodeLib/IGBT//Diode  Ron=1e-3  Rs=1e5  Cs=inf  Measurements=on
  IGBT/Diode1 : spsIGBTDiodeLib/IGBT//Diode  Ron=1e-3  Rs=1e5  Cs=inf  Measurements=on
  NOT1 : Logic  Operator=NOT  IconShape=distinctive  AllPortsSameDT=off  OutDataTypeStr=boolean
  Series RLC Branch2 : spsSeriesRLCBranchLib/Series RLC Branch  LConnTagsString=__new0  RConnTagsString=__new0  BranchType=C  Resistance=1  Inductance=1e-3  SetiL0=off  InitialCurrent=0  Capacitance=Cap  Setx0=on  InitialVoltage=Initial_Voltage  Measurements=Branch voltage and current
  + : PMIOPort  Side=Left
  - : PMIOPort  Port=2  Side=Right
  wires:
  Input/1 -> IGBT/Diode/1, NOT1/1
  NOT1/1 -> IGBT/Diode1/1
  connections:
  +/RConn1 -- IGBT/Diode1/LConn1 -- IGBT/Diode/RConn1
  Series RLC Branch2/LConn1 -- IGBT/Diode/LConn1
  Series RLC Branch2/RConn1 -- -/RConn1 -- IGBT/Diode1/RConn1

== system Voltage_Vector_with_script_fianl/3 ph 7 level MMI/SM 4 phase C ==
  Input : Inport
  IGBT/Diode : spsIGBTDiodeLib/IGBT//Diode  Ron=1e-3  Rs=1e5  Cs=inf  Measurements=on
  IGBT/Diode1 : spsIGBTDiodeLib/IGBT//Diode  Ron=1e-3  Rs=1e5  Cs=inf  Measurements=on
  NOT1 : Logic  Operator=NOT  IconShape=distinctive  AllPortsSameDT=off  OutDataTypeStr=boolean
  Series RLC Branch2 : spsSeriesRLCBranchLib/Series RLC Branch  LConnTagsString=__new0  RConnTagsString=__new0  BranchType=C  Resistance=1  Inductance=1e-3  SetiL0=off  InitialCurrent=0  Capacitance=Cap  Setx0=on  InitialVoltage=Initial_Voltage  Measurements=Branch voltage and current
  + : PMIOPort  Side=Left
  - : PMIOPort  Port=2  Side=Right
  wires:
  Input/1 -> IGBT/Diode/1, NOT1/1
  NOT1/1 -> IGBT/Diode1/1
  connections:
  +/RConn1 -- IGBT/Diode1/LConn1 -- IGBT/Diode/RConn1
  Series RLC Branch2/LConn1 -- IGBT/Diode/LConn1
  Series RLC Branch2/RConn1 -- -/RConn1 -- IGBT/Diode1/RConn1

== system Voltage_Vector_with_script_fianl/3 ph 7 level MMI/SM 5 phase A ==
  Input : Inport
  IGBT/Diode : spsIGBTDiodeLib/IGBT//Diode  Ron=1e-3  Rs=1e5  Cs=inf  Measurements=on
  IGBT/Diode1 : spsIGBTDiodeLib/IGBT//Diode  Ron=1e-3  Rs=1e5  Cs=inf  Measurements=on
  NOT1 : Logic  Operator=NOT  IconShape=distinctive  AllPortsSameDT=off  OutDataTypeStr=boolean
  Series RLC Branch2 : spsSeriesRLCBranchLib/Series RLC Branch  LConnTagsString=__new0  RConnTagsString=__new0  BranchType=C  Resistance=1  Inductance=1e-3  SetiL0=off  InitialCurrent=0  Capacitance=Cap  Setx0=on  InitialVoltage=Initial_Voltage  Measurements=Branch voltage and current
  + : PMIOPort  Side=Left
  - : PMIOPort  Port=2  Side=Right
  wires:
  Input/1 -> IGBT/Diode/1, NOT1/1
  NOT1/1 -> IGBT/Diode1/1
  connections:
  +/RConn1 -- IGBT/Diode1/LConn1 -- IGBT/Diode/RConn1
  Series RLC Branch2/LConn1 -- IGBT/Diode/LConn1
  Series RLC Branch2/RConn1 -- -/RConn1 -- IGBT/Diode1/RConn1

== system Voltage_Vector_with_script_fianl/3 ph 7 level MMI/SM 5 phase B ==
  Input : Inport
  IGBT/Diode : spsIGBTDiodeLib/IGBT//Diode  Ron=1e-3  Rs=1e5  Cs=inf  Measurements=on
  IGBT/Diode1 : spsIGBTDiodeLib/IGBT//Diode  Ron=1e-3  Rs=1e5  Cs=inf  Measurements=on
  NOT1 : Logic  Operator=NOT  IconShape=distinctive  AllPortsSameDT=off  OutDataTypeStr=boolean
  Series RLC Branch2 : spsSeriesRLCBranchLib/Series RLC Branch  LConnTagsString=__new0  RConnTagsString=__new0  BranchType=C  Resistance=1  Inductance=1e-3  SetiL0=off  InitialCurrent=0  Capacitance=Cap  Setx0=on  InitialVoltage=Initial_Voltage  Measurements=Branch voltage and current
  + : PMIOPort  Side=Left
  - : PMIOPort  Port=2  Side=Right
  wires:
  Input/1 -> IGBT/Diode/1, NOT1/1
  NOT1/1 -> IGBT/Diode1/1
  connections:
  +/RConn1 -- IGBT/Diode1/LConn1 -- IGBT/Diode/RConn1
  Series RLC Branch2/LConn1 -- IGBT/Diode/LConn1
  Series RLC Branch2/RConn1 -- -/RConn1 -- IGBT/Diode1/RConn1

== system Voltage_Vector_with_script_fianl/3 ph 7 level MMI/SM 5 phase C ==
  Input : Inport
  IGBT/Diode : spsIGBTDiodeLib/IGBT//Diode  Ron=1e-3  Rs=1e5  Cs=inf  Measurements=on
  IGBT/Diode1 : spsIGBTDiodeLib/IGBT//Diode  Ron=1e-3  Rs=1e5  Cs=inf  Measurements=on
  NOT1 : Logic  Operator=NOT  IconShape=distinctive  AllPortsSameDT=off  OutDataTypeStr=boolean
  Series RLC Branch2 : spsSeriesRLCBranchLib/Series RLC Branch  LConnTagsString=__new0  RConnTagsString=__new0  BranchType=C  Resistance=1  Inductance=1e-3  SetiL0=off  InitialCurrent=0  Capacitance=Cap  Setx0=on  InitialVoltage=Initial_Voltage  Measurements=Branch voltage and current
  + : PMIOPort  Side=Left
  - : PMIOPort  Port=2  Side=Right
  wires:
  Input/1 -> IGBT/Diode/1, NOT1/1
  NOT1/1 -> IGBT/Diode1/1
  connections:
  +/RConn1 -- IGBT/Diode1/LConn1 -- IGBT/Diode/RConn1
  Series RLC Branch2/LConn1 -- IGBT/Diode/LConn1
  Series RLC Branch2/RConn1 -- -/RConn1 -- IGBT/Diode1/RConn1

== system Voltage_Vector_with_script_fianl/3 ph 7 level MMI/SM 6 phase A ==
  Input : Inport
  IGBT/Diode : spsIGBTDiodeLib/IGBT//Diode  Ron=1e-3  Rs=1e5  Cs=inf  Measurements=on
  IGBT/Diode1 : spsIGBTDiodeLib/IGBT//Diode  Ron=1e-3  Rs=1e5  Cs=inf  Measurements=on
  NOT1 : Logic  Operator=NOT  IconShape=distinctive  AllPortsSameDT=off  OutDataTypeStr=boolean
  Scope : Scope
  Series RLC Branch2 : spsSeriesRLCBranchLib/Series RLC Branch  LConnTagsString=__new0  RConnTagsString=__new0  BranchType=C  Resistance=1  Inductance=1e-3  SetiL0=off  InitialCurrent=0  Capacitance=Cap  Setx0=on  InitialVoltage=Initial_Voltage  Measurements=Branch voltage and current
  + : PMIOPort  Side=Left
  - : PMIOPort  Port=2  Side=Right
  wires:
  Input/1 -> Scope/1, IGBT/Diode/1, NOT1/1
  NOT1/1 -> IGBT/Diode1/1
  connections:
  +/RConn1 -- IGBT/Diode1/LConn1 -- IGBT/Diode/RConn1
  Series RLC Branch2/LConn1 -- IGBT/Diode/LConn1
  Series RLC Branch2/RConn1 -- -/RConn1 -- IGBT/Diode1/RConn1

== system Voltage_Vector_with_script_fianl/3 ph 7 level MMI/SM 6 phase B ==
  Input : Inport
  IGBT/Diode : spsIGBTDiodeLib/IGBT//Diode  Ron=1e-3  Rs=1e5  Cs=inf  Measurements=on
  IGBT/Diode1 : spsIGBTDiodeLib/IGBT//Diode  Ron=1e-3  Rs=1e5  Cs=inf  Measurements=on
  NOT1 : Logic  Operator=NOT  IconShape=distinctive  AllPortsSameDT=off  OutDataTypeStr=boolean
  Series RLC Branch2 : spsSeriesRLCBranchLib/Series RLC Branch  LConnTagsString=__new0  RConnTagsString=__new0  BranchType=C  Resistance=1  Inductance=1e-3  SetiL0=off  InitialCurrent=0  Capacitance=Cap  Setx0=on  InitialVoltage=Initial_Voltage  Measurements=Branch voltage and current
  + : PMIOPort  Side=Left
  - : PMIOPort  Port=2  Side=Right
  wires:
  Input/1 -> IGBT/Diode/1, NOT1/1
  NOT1/1 -> IGBT/Diode1/1
  connections:
  +/RConn1 -- IGBT/Diode1/LConn1 -- IGBT/Diode/RConn1
  Series RLC Branch2/LConn1 -- IGBT/Diode/LConn1
  Series RLC Branch2/RConn1 -- -/RConn1 -- IGBT/Diode1/RConn1

== system Voltage_Vector_with_script_fianl/3 ph 7 level MMI/SM 6 phase C ==
  Input : Inport
  IGBT/Diode : spsIGBTDiodeLib/IGBT//Diode  Ron=1e-3  Rs=1e5  Cs=inf  Measurements=on
  IGBT/Diode1 : spsIGBTDiodeLib/IGBT//Diode  Ron=1e-3  Rs=1e5  Cs=inf  Measurements=on
  NOT1 : Logic  Operator=NOT  IconShape=distinctive  AllPortsSameDT=off  OutDataTypeStr=boolean
  Series RLC Branch2 : spsSeriesRLCBranchLib/Series RLC Branch  LConnTagsString=__new0  RConnTagsString=__new0  BranchType=C  Resistance=1  Inductance=1e-3  SetiL0=off  InitialCurrent=0  Capacitance=Cap  Setx0=on  InitialVoltage=Initial_Voltage  Measurements=Branch voltage and current
  + : PMIOPort  Side=Left
  - : PMIOPort  Port=2  Side=Right
  wires:
  Input/1 -> IGBT/Diode/1, NOT1/1
  NOT1/1 -> IGBT/Diode1/1
  connections:
  +/RConn1 -- IGBT/Diode1/LConn1 -- IGBT/Diode/RConn1
  Series RLC Branch2/LConn1 -- IGBT/Diode/LConn1
  Series RLC Branch2/RConn1 -- -/RConn1 -- IGBT/Diode1/RConn1

== system Voltage_Vector_with_script_fianl/3 ph 7 level MMI/SM 7 phase A ==
  Input : Inport
  IGBT/Diode : spsIGBTDiodeLib/IGBT//Diode  Ron=1e-3  Rs=1e5  Cs=inf  Measurements=on
  IGBT/Diode1 : spsIGBTDiodeLib/IGBT//Diode  Ron=1e-3  Rs=1e5  Cs=inf  Measurements=on
  NOT1 : Logic  Operator=NOT  IconShape=distinctive  AllPortsSameDT=off  OutDataTypeStr=boolean
  Series RLC Branch2 : spsSeriesRLCBranchLib/Series RLC Branch  LConnTagsString=__new0  RConnTagsString=__new0  BranchType=C  Resistance=1  Inductance=1e-3  SetiL0=off  InitialCurrent=0  Capacitance=Cap  Setx0=on  InitialVoltage=Initial_Voltage  Measurements=Branch voltage and current
  + : PMIOPort  Side=Left
  - : PMIOPort  Port=2  Side=Right
  wires:
  Input/1 -> IGBT/Diode/1, NOT1/1
  NOT1/1 -> IGBT/Diode1/1
  connections:
  +/RConn1 -- IGBT/Diode1/LConn1 -- IGBT/Diode/RConn1
  Series RLC Branch2/LConn1 -- IGBT/Diode/LConn1
  Series RLC Branch2/RConn1 -- -/RConn1 -- IGBT/Diode1/RConn1

== system Voltage_Vector_with_script_fianl/3 ph 7 level MMI/SM 7 phase B ==
  Input : Inport
  IGBT/Diode : spsIGBTDiodeLib/IGBT//Diode  Ron=1e-3  Rs=1e5  Cs=inf  Measurements=on
  IGBT/Diode1 : spsIGBTDiodeLib/IGBT//Diode  Ron=1e-3  Rs=1e5  Cs=inf  Measurements=on
  NOT1 : Logic  Operator=NOT  IconShape=distinctive  AllPortsSameDT=off  OutDataTypeStr=boolean
  Series RLC Branch2 : spsSeriesRLCBranchLib/Series RLC Branch  LConnTagsString=__new0  RConnTagsString=__new0  BranchType=C  Resistance=1  Inductance=1e-3  SetiL0=off  InitialCurrent=0  Capacitance=Cap  Setx0=on  InitialVoltage=Initial_Voltage  Measurements=Branch voltage and current
  + : PMIOPort  Side=Left
  - : PMIOPort  Port=2  Side=Right
  wires:
  Input/1 -> IGBT/Diode/1, NOT1/1
  NOT1/1 -> IGBT/Diode1/1
  connections:
  +/RConn1 -- IGBT/Diode1/LConn1 -- IGBT/Diode/RConn1
  Series RLC Branch2/LConn1 -- IGBT/Diode/LConn1
  Series RLC Branch2/RConn1 -- -/RConn1 -- IGBT/Diode1/RConn1

== system Voltage_Vector_with_script_fianl/3 ph 7 level MMI/SM 7 phase C ==
  Input : Inport
  IGBT/Diode : spsIGBTDiodeLib/IGBT//Diode  Ron=1e-3  Rs=1e5  Cs=inf  Measurements=on
  IGBT/Diode1 : spsIGBTDiodeLib/IGBT//Diode  Ron=1e-3  Rs=1e5  Cs=inf  Measurements=on
  NOT1 : Logic  Operator=NOT  IconShape=distinctive  AllPortsSameDT=off  OutDataTypeStr=boolean
  Series RLC Branch2 : spsSeriesRLCBranchLib/Series RLC Branch  LConnTagsString=__new0  RConnTagsString=__new0  BranchType=C  Resistance=1  Inductance=1e-3  SetiL0=off  InitialCurrent=0  Capacitance=Cap  Setx0=on  InitialVoltage=Initial_Voltage  Measurements=Branch voltage and current
  + : PMIOPort  Side=Left
  - : PMIOPort  Port=2  Side=Right
  wires:
  Input/1 -> IGBT/Diode/1, NOT1/1
  NOT1/1 -> IGBT/Diode1/1
  connections:
  +/RConn1 -- IGBT/Diode1/LConn1 -- IGBT/Diode/RConn1
  Series RLC Branch2/LConn1 -- IGBT/Diode/LConn1
  Series RLC Branch2/RConn1 -- -/RConn1 -- IGBT/Diode1/RConn1

== system Voltage_Vector_with_script_fianl/3 ph 7 level MMI/SM 8 phase A ==
  Input : Inport
  IGBT/Diode : spsIGBTDiodeLib/IGBT//Diode  Ron=1e-3  Rs=1e5  Cs=inf  Measurements=on
  IGBT/Diode1 : spsIGBTDiodeLib/IGBT//Diode  Ron=1e-3  Rs=1e5  Cs=inf  Measurements=on
  NOT1 : Logic  Operator=NOT  IconShape=distinctive  AllPortsSameDT=off  OutDataTypeStr=boolean
  Series RLC Branch2 : spsSeriesRLCBranchLib/Series RLC Branch  LConnTagsString=__new0  RConnTagsString=__new0  BranchType=C  Resistance=1  Inductance=1e-3  SetiL0=off  InitialCurrent=0  Capacitance=Cap  Setx0=on  InitialVoltage=Initial_Voltage  Measurements=Branch voltage and current
  + : PMIOPort  Side=Left
  - : PMIOPort  Port=2  Side=Right
  wires:
  Input/1 -> IGBT/Diode/1, NOT1/1
  NOT1/1 -> IGBT/Diode1/1
  connections:
  +/RConn1 -- IGBT/Diode1/LConn1 -- IGBT/Diode/RConn1
  Series RLC Branch2/LConn1 -- IGBT/Diode/LConn1
  Series RLC Branch2/RConn1 -- -/RConn1 -- IGBT/Diode1/RConn1

== system Voltage_Vector_with_script_fianl/3 ph 7 level MMI/SM 8 phase B ==
  Input : Inport
  IGBT/Diode : spsIGBTDiodeLib/IGBT//Diode  Ron=1e-3  Rs=1e5  Cs=inf  Measurements=on
  IGBT/Diode1 : spsIGBTDiodeLib/IGBT//Diode  Ron=1e-3  Rs=1e5  Cs=inf  Measurements=on
  NOT1 : Logic  Operator=NOT  IconShape=distinctive  AllPortsSameDT=off  OutDataTypeStr=boolean
  Series RLC Branch2 : spsSeriesRLCBranchLib/Series RLC Branch  LConnTagsString=__new0  RConnTagsString=__new0  BranchType=C  Resistance=1  Inductance=1e-3  SetiL0=off  InitialCurrent=0  Capacitance=Cap  Setx0=on  InitialVoltage=Initial_Voltage  Measurements=Branch voltage and current
  + : PMIOPort  Side=Left
  - : PMIOPort  Port=2  Side=Right
  wires:
  Input/1 -> IGBT/Diode/1, NOT1/1
  NOT1/1 -> IGBT/Diode1/1
  connections:
  +/RConn1 -- IGBT/Diode1/LConn1 -- IGBT/Diode/RConn1
  Series RLC Branch2/LConn1 -- IGBT/Diode/LConn1
  Series RLC Branch2/RConn1 -- -/RConn1 -- IGBT/Diode1/RConn1

== system Voltage_Vector_with_script_fianl/3 ph 7 level MMI/SM 8 phase C ==
  Input : Inport
  IGBT/Diode : spsIGBTDiodeLib/IGBT//Diode  Ron=1e-3  Rs=1e5  Cs=inf  Measurements=on
  IGBT/Diode1 : spsIGBTDiodeLib/IGBT//Diode  Ron=1e-3  Rs=1e5  Cs=inf  Measurements=on
  NOT1 : Logic  Operator=NOT  IconShape=distinctive  AllPortsSameDT=off  OutDataTypeStr=boolean
  Series RLC Branch2 : spsSeriesRLCBranchLib/Series RLC Branch  LConnTagsString=__new0  RConnTagsString=__new0  BranchType=C  Resistance=1  Inductance=1e-3  SetiL0=off  InitialCurrent=0  Capacitance=Cap  Setx0=on  InitialVoltage=Initial_Voltage  Measurements=Branch voltage and current
  + : PMIOPort  Side=Left
  - : PMIOPort  Port=2  Side=Right
  wires:
  Input/1 -> IGBT/Diode/1, NOT1/1
  NOT1/1 -> IGBT/Diode1/1
  connections:
  +/RConn1 -- IGBT/Diode1/LConn1 -- IGBT/Diode/RConn1
  Series RLC Branch2/LConn1 -- IGBT/Diode/LConn1
  Series RLC Branch2/RConn1 -- -/RConn1 -- IGBT/Diode1/RConn1

== system Voltage_Vector_with_script_fianl/3 ph 7 level MMI/SM 9 phase A ==
  Input : Inport
  IGBT/Diode : spsIGBTDiodeLib/IGBT//Diode  Ron=1e-3  Rs=1e5  Cs=inf  Measurements=on
  IGBT/Diode1 : spsIGBTDiodeLib/IGBT//Diode  Ron=1e-3  Rs=1e5  Cs=inf  Measurements=on
  NOT1 : Logic  Operator=NOT  IconShape=distinctive  AllPortsSameDT=off  OutDataTypeStr=boolean
  Series RLC Branch2 : spsSeriesRLCBranchLib/Series RLC Branch  LConnTagsString=__new0  RConnTagsString=__new0  BranchType=C  Resistance=1  Inductance=1e-3  SetiL0=off  InitialCurrent=0  Capacitance=Cap  Setx0=on  InitialVoltage=Initial_Voltage  Measurements=Branch voltage and current
  + : PMIOPort  Side=Left
  - : PMIOPort  Port=2  Side=Right
  wires:
  Input/1 -> IGBT/Diode/1, NOT1/1
  NOT1/1 -> IGBT/Diode1/1
  connections:
  +/RConn1 -- IGBT/Diode1/LConn1 -- IGBT/Diode/RConn1
  Series RLC Branch2/LConn1 -- IGBT/Diode/LConn1
  Series RLC Branch2/RConn1 -- -/RConn1 -- IGBT/Diode1/RConn1

== system Voltage_Vector_with_script_fianl/3 ph 7 level MMI/SM 9 phase B ==
  Input : Inport
  IGBT/Diode : spsIGBTDiodeLib/IGBT//Diode  Ron=1e-3  Rs=1e5  Cs=inf  Measurements=on
  IGBT/Diode1 : spsIGBTDiodeLib/IGBT//Diode  Ron=1e-3  Rs=1e5  Cs=inf  Measurements=on
  NOT1 : Logic  Operator=NOT  IconShape=distinctive  AllPortsSameDT=off  OutDataTypeStr=boolean
  Series RLC Branch2 : spsSeriesRLCBranchLib/Series RLC Branch  LConnTagsString=__new0  RConnTagsString=__new0  BranchType=C  Resistance=1  Inductance=1e-3  SetiL0=off  InitialCurrent=0  Capacitance=Cap  Setx0=on  InitialVoltage=Initial_Voltage  Measurements=Branch voltage and current
  + : PMIOPort  Side=Left
  - : PMIOPort  Port=2  Side=Right
  wires:
  Input/1 -> IGBT/Diode/1, NOT1/1
  NOT1/1 -> IGBT/Diode1/1
  connections:
  +/RConn1 -- IGBT/Diode1/LConn1 -- IGBT/Diode/RConn1
  Series RLC Branch2/LConn1 -- IGBT/Diode/LConn1
  Series RLC Branch2/RConn1 -- -/RConn1 -- IGBT/Diode1/RConn1

== system Voltage_Vector_with_script_fianl/3 ph 7 level MMI/SM 9 phase C ==
  Input : Inport
  IGBT/Diode : spsIGBTDiodeLib/IGBT//Diode  Ron=1e-3  Rs=1e5  Cs=inf  Measurements=on
  IGBT/Diode1 : spsIGBTDiodeLib/IGBT//Diode  Ron=1e-3  Rs=1e5  Cs=inf  Measurements=on
  NOT1 : Logic  Operator=NOT  IconShape=distinctive  AllPortsSameDT=off  OutDataTypeStr=boolean
  Series RLC Branch2 : spsSeriesRLCBranchLib/Series RLC Branch  LConnTagsString=__new0  RConnTagsString=__new0  BranchType=C  Resistance=1  Inductance=1e-3  SetiL0=off  InitialCurrent=0  Capacitance=Cap  Setx0=on  InitialVoltage=Initial_Voltage  Measurements=Branch voltage and current
  + : PMIOPort  Side=Left
  - : PMIOPort  Port=2  Side=Right
  wires:
  Input/1 -> IGBT/Diode/1, NOT1/1
  NOT1/1 -> IGBT/Diode1/1
  connections:
  +/RConn1 -- IGBT/Diode1/LConn1 -- IGBT/Diode/RConn1
  Series RLC Branch2/LConn1 -- IGBT/Diode/LConn1
  Series RLC Branch2/RConn1 -- -/RConn1 -- IGBT/Diode1/RConn1

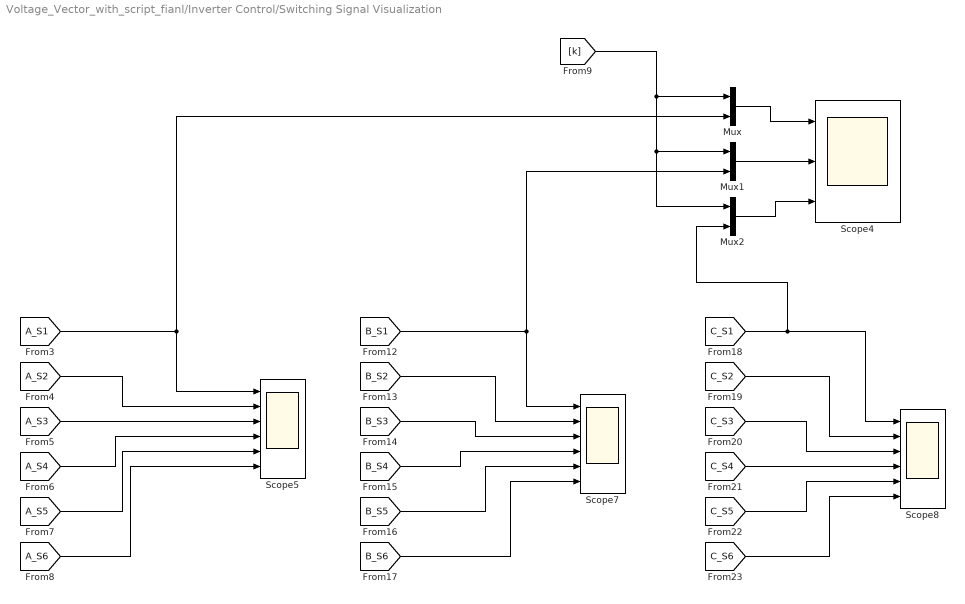
== system Voltage_Vector_with_script_fianl/Inverter Control/Switching Signal Visualization ==
  Mux : Mux  Inputs=2
  Mux1 : Mux  Inputs=2
  Mux2 : Mux  Inputs=2
  Scope4 : Scope  NumInputPorts=3
  Scope5 : Scope  NumInputPorts=6
  Scope7 : Scope  NumInputPorts=6
  Scope8 : Scope  NumInputPorts=6
  wires:
  [A_S1] -> Mux/2, Scope5/1
  [C_S4] -> Scope8/4
  [C_S5] -> Scope8/5
  [A_S6] -> Scope5/6
  [B_S4] -> Scope7/4
  [C_S2] -> Scope8/2
  [B_S6] -> Scope7/6
  [A_S3] -> Scope5/3
  [B_S1] -> Mux1/2, Scope7/1
  [B_S2] -> Scope7/2
  [k] -> Mux/1, Mux1/1, Mux2/1
  [A_S5] -> Scope5/5
  [A_S2] -> Scope5/2
  [B_S3] -> Scope7/3
  [A_S4] -> Scope5/4
  [C_S3] -> Scope8/3
  [C_S1] -> Mux2/2, Scope8/1
  [B_S5] -> Scope7/5
  [C_S6] -> Scope8/6
  Mux/1 -> Scope4/1
  Mux1/1 -> Scope4/2
  Mux2/1 -> Scope4/3
